simulink library "tramontina_database_RCU_Comissionamentolib"  (R2024a)
settings: Solver=VariableStepAuto  StartTime=0.0  StopTime=10.0  RelTol=1e-3
libraries: canmsglib x4, simulink x1
settings Model: Creator=matlab.cut  LastModifiedBy=matlab.cut

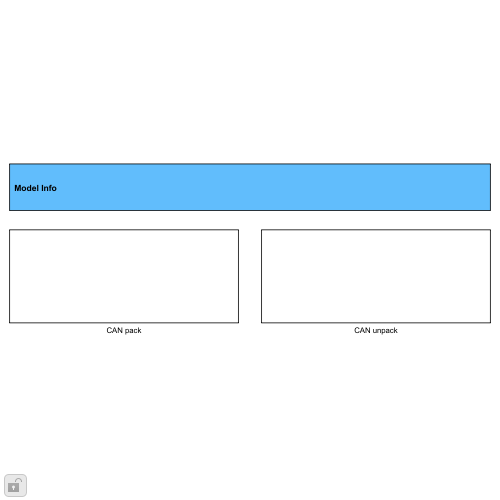
[thumbnail: Simulink's stored preview of the top-level diagram]
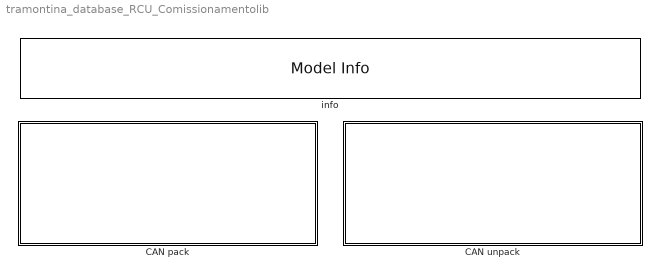
== system tramontina_database_RCU_Comissionamentolib ==
  CAN pack : Subsystem
  CAN unpack : Subsystem
  info : simulink/Model-Wide Utilities/Model Info  Frame=on  DisplayStringWithTags=SPEEDGOAT CAN Database Library for: tramontina_database_RCU_Comissionamento  HorizontalTextAlignment=Left  LeftAlignmentValue=0.01

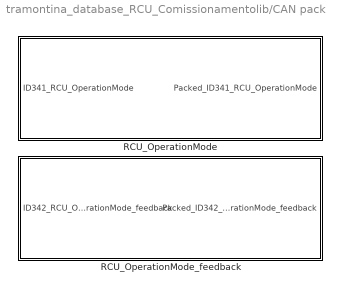
== system tramontina_database_RCU_Comissionamentolib/CAN pack ==
  RCU_OperationMode : Subsystem
  RCU_OperationMode_feedback : Subsystem

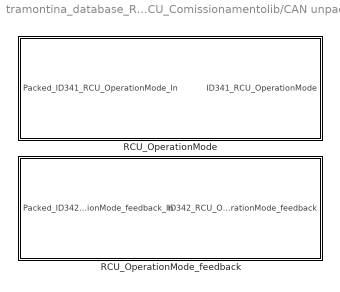
== system tramontina_database_RCU_Comissionamentolib/CAN unpack ==
  RCU_OperationMode : Subsystem
  RCU_OperationMode_feedback : Subsystem

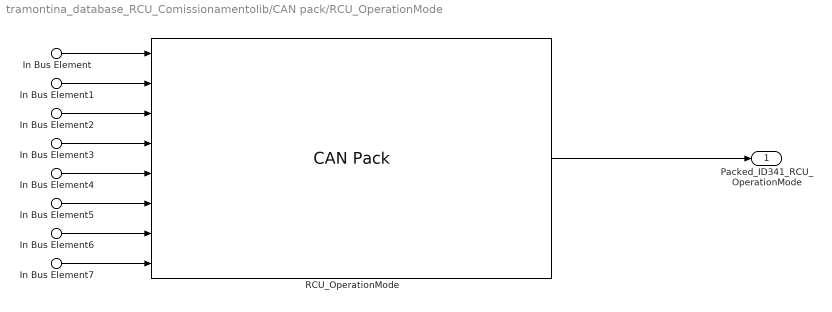
== system tramontina_database_RCU_Comissionamentolib/CAN pack/RCU_OperationMode ==
  In Bus Element : Inport  PortName=ID341_RCU_OperationMode  Element=rcu_front_LeftRigth
  In Bus Element1 : Inport  PortName=ID341_RCU_OperationMode  Element=rcu_front_LoadUnload
  In Bus Element2 : Inport  PortName=ID341_RCU_OperationMode  Element=rcu_front_Run
  In Bus Element3 : Inport  PortName=ID341_RCU_OperationMode  Element=rcu_front_isMoving
  In Bus Element4 : Inport  PortName=ID341_RCU_OperationMode  Element=rcu_rear_LeftRigth
  In Bus Element5 : Inport  PortName=ID341_RCU_OperationMode  Element=rcu_rear_LoadUnload
  In Bus Element6 : Inport  PortName=ID341_RCU_OperationMode  Element=rcu_rear_Run
  In Bus Element7 : Inport  PortName=ID341_RCU_OperationMode  Element=rcu_rear_isMoving
  RCU_OperationMode : canmsglib/CAN Pack  CANdbFile=C:\Users\matlab.cut\Desktop\matlab\AMR_tramontina\Data\DBCFiles\tramontina_database_RCU_Comissionamento.dbc  MsgList=RCU_OperationMode  MsgName=RCU_OperationMode  MsgIDType=Standard (11-bit identifier)  MsgIdentifier=341  MsgLength=8  Remote=off  ApplyMinMax=off  BusOutput=on  SignalInfo={'rcu_front_LeftRigth','1','1','LE','unsigned','Standard','0','1','0','-Inf','Inf';'rcu_front_LoadUnload','0','1','LE','unsigned','Standard','0','1','0','-Inf','Inf';'rcu_front_Run','2','1','LE','unsigned','Standard','0','1','0','-Inf','Inf';'rcu_front_isMoving','3','1','LE','unsigned','Standard','0','1','0','-Inf','Inf';'rcu_rear_LeftRigth','9','1','LE','unsigned','Standard','0','1','0','-Inf','Inf';'rcu_rear_LoadUnload','8','1','LE','unsigned','Standard','0','1','0','-Inf','Inf';'rcu_rear_Run','10','1','LE','unsigned','Standard','0','1','0','-Inf','Inf';'rcu_rear_isMoving','11','1','LE','unsigned','Standard','0','1','0','-Inf','Inf'}
      settings: DataFormat=manually specified signals
  Packed_ID341_RCU_OperationMode : Outport
  wires:
  RCU_OperationMode/1 -> Packed_ID341_RCU_OperationMode/1
  In Bus Element/1 -> RCU_OperationMode/1
  In Bus Element1/1 -> RCU_OperationMode/2
  In Bus Element2/1 -> RCU_OperationMode/3
  In Bus Element3/1 -> RCU_OperationMode/4
  In Bus Element4/1 -> RCU_OperationMode/5
  In Bus Element5/1 -> RCU_OperationMode/6
  In Bus Element6/1 -> RCU_OperationMode/7
  In Bus Element7/1 -> RCU_OperationMode/8

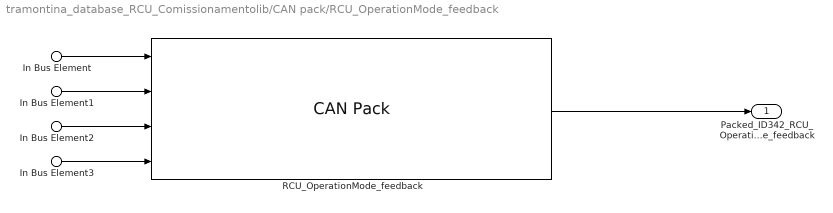
== system tramontina_database_RCU_Comissionamentolib/CAN pack/RCU_OperationMode_feedback ==
  In Bus Element : Inport  PortName=ID342_RCU_OperationMode_feedback  Element=rcu_front_LeftRigth_feedback
  In Bus Element1 : Inport  PortName=ID342_RCU_OperationMode_feedback  Element=rcu_front_LoadUnload_feedback
  In Bus Element2 : Inport  PortName=ID342_RCU_OperationMode_feedback  Element=rcu_front_Run_feedback
  In Bus Element3 : Inport  PortName=ID342_RCU_OperationMode_feedback  Element=rcu_front_isMoving_feedback
  RCU_OperationMode_feedback : canmsglib/CAN Pack  CANdbFile=C:\Users\matlab.cut\Desktop\matlab\AMR_tramontina\Data\DBCFiles\tramontina_database_RCU_Comissionamento.dbc  MsgList=RCU_OperationMode_feedback  MsgName=RCU_OperationMode_feedback  MsgIDType=Standard (11-bit identifier)  MsgIdentifier=342  MsgLength=8  Remote=off  ApplyMinMax=off  BusOutput=on  SignalInfo={'rcu_front_LeftRigth_feedback','1','1','LE','unsigned','Standard','0','1','0','-Inf','Inf';'rcu_front_LoadUnload_feedback','0','1','LE','unsigned','Standard','0','1','0','-Inf','Inf';'rcu_front_Run_feedback','2','1','LE','unsigned','Standard','0','1','0','-Inf','Inf';'rcu_front_isMoving_feedback','3','1','LE','unsigned','Standard','0','1','0','-Inf','Inf'}
      settings: DataFormat=manually specified signals
  Packed_ID342_RCU_OperationMode_feedback : Outport
  wires:
  RCU_OperationMode_feedback/1 -> Packed_ID342_RCU_OperationMode_feedback/1
  In Bus Element/1 -> RCU_OperationMode_feedback/1
  In Bus Element1/1 -> RCU_OperationMode_feedback/2
  In Bus Element2/1 -> RCU_OperationMode_feedback/3
  In Bus Element3/1 -> RCU_OperationMode_feedback/4

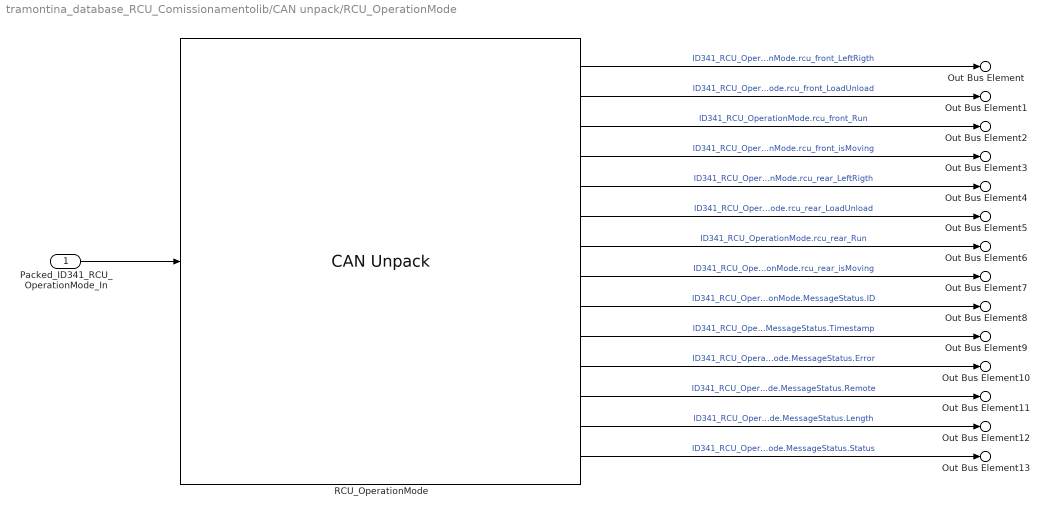
== system tramontina_database_RCU_Comissionamentolib/CAN unpack/RCU_OperationMode ==
  Packed_ID341_RCU_OperationMode_In : Inport
  RCU_OperationMode : canmsglib/CAN Unpack  CANdbFile=C:\Users\matlab.cut\Desktop\matlab\AMR_tramontina\Data\DBCFiles\tramontina_database_RCU_Comissionamento.dbc  MsgList=RCU_OperationMode  MsgName=RCU_OperationMode  MsgIDType=Standard (11-bit identifier)  MsgIdentifier=341  MsgLength=8  SignalInfo={'rcu_front_LeftRigth','1','1','LE','unsigned','Standard','0','1','0','-Inf','Inf';'rcu_front_LoadUnload','0','1','LE','unsigned','Standard','0','1','0','-Inf','Inf';'rcu_front_Run','2','1','LE','unsigned','Standard','0','1','0','-Inf','Inf';'rcu_front_isMoving','3','1','LE','unsigned','Standard','0','1','0','-Inf','Inf';'rcu_rear_LeftRigth','9','1','LE','unsigned','Standard','0','1','0','-Inf','Inf';'rcu_rear_LoadUnload','8','1','LE','unsigned','Standard','0','1','0','-Inf','Inf';'rcu_rear_Run','10','1','LE','unsigned','Standard','0','1','0','-Inf','Inf';'rcu_rear_isMoving','11','1','LE','unsigned','Standard','0','1','0','-Inf','Inf'}  IDPort=on  TimestampPort=on  ErrorPort=on  RemotePort=on  LengthPort=on  StatusPort=on  ApplyMinMax=off
  Out Bus Element : Outport  PortName=ID341_RCU_OperationMode  Element=rcu_front_LeftRigth
  Out Bus Element1 : Outport  PortName=ID341_RCU_OperationMode  Element=rcu_front_LoadUnload
  Out Bus Element2 : Outport  PortName=ID341_RCU_OperationMode  Element=rcu_front_Run
  Out Bus Element3 : Outport  PortName=ID341_RCU_OperationMode  Element=rcu_front_isMoving
  Out Bus Element4 : Outport  PortName=ID341_RCU_OperationMode  Element=rcu_rear_LeftRigth
  Out Bus Element5 : Outport  PortName=ID341_RCU_OperationMode  Element=rcu_rear_LoadUnload
  Out Bus Element6 : Outport  PortName=ID341_RCU_OperationMode  Element=rcu_rear_Run
  Out Bus Element7 : Outport  PortName=ID341_RCU_OperationMode  Element=rcu_rear_isMoving
  Out Bus Element8 : Outport  PortName=ID341_RCU_OperationMode  Element=MessageStatus.ID
  Out Bus Element9 : Outport  PortName=ID341_RCU_OperationMode  Element=MessageStatus.Timestamp
  Out Bus Element10 : Outport  PortName=ID341_RCU_OperationMode  Element=MessageStatus.Error
  Out Bus Element11 : Outport  PortName=ID341_RCU_OperationMode  Element=MessageStatus.Remote
  Out Bus Element12 : Outport  PortName=ID341_RCU_OperationMode  Element=MessageStatus.Length
  Out Bus Element13 : Outport  PortName=ID341_RCU_OperationMode  Element=MessageStatus.Status
  wires:
  Packed_ID341_RCU_OperationMode_In/1 -> RCU_OperationMode/1
  RCU_OperationMode/1 -> Out Bus Element/1  "ID341_RCU_OperationMode.rcu_front_LeftRigth"
  RCU_OperationMode/2 -> Out Bus Element1/1  "ID341_RCU_OperationMode.rcu_front_LoadUnload"
  RCU_OperationMode/3 -> Out Bus Element2/1  "ID341_RCU_OperationMode.rcu_front_Run"
  RCU_OperationMode/4 -> Out Bus Element3/1  "ID341_RCU_OperationMode.rcu_front_isMoving"
  RCU_OperationMode/5 -> Out Bus Element4/1  "ID341_RCU_OperationMode.rcu_rear_LeftRigth"
  RCU_OperationMode/6 -> Out Bus Element5/1  "ID341_RCU_OperationMode.rcu_rear_LoadUnload"
  RCU_OperationMode/7 -> Out Bus Element6/1  "ID341_RCU_OperationMode.rcu_rear_Run"
  RCU_OperationMode/8 -> Out Bus Element7/1  "ID341_RCU_OperationMode.rcu_rear_isMoving"
  RCU_OperationMode/9 -> Out Bus Element8/1  "ID341_RCU_OperationMode.MessageStatus.ID"
  RCU_OperationMode/10 -> Out Bus Element9/1  "ID341_RCU_OperationMode.MessageStatus.Timestamp"
  RCU_OperationMode/11 -> Out Bus Element10/1  "ID341_RCU_OperationMode.MessageStatus.Error"
  RCU_OperationMode/12 -> Out Bus Element11/1  "ID341_RCU_OperationMode.MessageStatus.Remote"
  RCU_OperationMode/13 -> Out Bus Element12/1  "ID341_RCU_OperationMode.MessageStatus.Length"
  RCU_OperationMode/14 -> Out Bus Element13/1  "ID341_RCU_OperationMode.MessageStatus.Status"

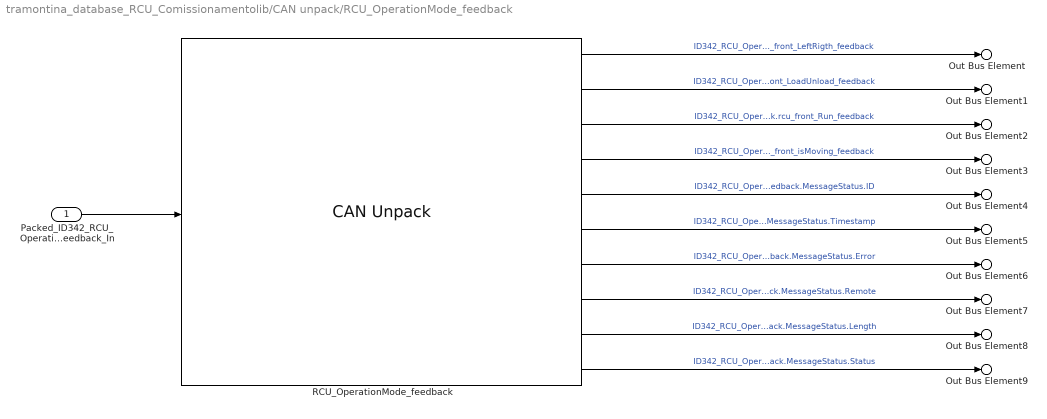
== system tramontina_database_RCU_Comissionamentolib/CAN unpack/RCU_OperationMode_feedback ==
  Packed_ID342_RCU_OperationMode_feedback_In : Inport
  RCU_OperationMode_feedback : canmsglib/CAN Unpack  CANdbFile=C:\Users\matlab.cut\Desktop\matlab\AMR_tramontina\Data\DBCFiles\tramontina_database_RCU_Comissionamento.dbc  MsgList=RCU_OperationMode_feedback  MsgName=RCU_OperationMode_feedback  MsgIDType=Standard (11-bit identifier)  MsgIdentifier=342  MsgLength=8  SignalInfo={'rcu_front_LeftRigth_feedback','1','1','LE','unsigned','Standard','0','1','0','-Inf','Inf';'rcu_front_LoadUnload_feedback','0','1','LE','unsigned','Standard','0','1','0','-Inf','Inf';'rcu_front_Run_feedback','2','1','LE','unsigned','Standard','0','1','0','-Inf','Inf';'rcu_front_isMoving_feedback','3','1','LE','unsigned','Standard','0','1','0','-Inf','Inf'}  IDPort=on  TimestampPort=on  ErrorPort=on  RemotePort=on  LengthPort=on  StatusPort=on  ApplyMinMax=off
  Out Bus Element : Outport  PortName=ID342_RCU_OperationMode_feedback  Element=rcu_front_LeftRigth_feedback
  Out Bus Element1 : Outport  PortName=ID342_RCU_OperationMode_feedback  Element=rcu_front_LoadUnload_feedback
  Out Bus Element2 : Outport  PortName=ID342_RCU_OperationMode_feedback  Element=rcu_front_Run_feedback
  Out Bus Element3 : Outport  PortName=ID342_RCU_OperationMode_feedback  Element=rcu_front_isMoving_feedback
  Out Bus Element4 : Outport  PortName=ID342_RCU_OperationMode_feedback  Element=MessageStatus.ID
  Out Bus Element5 : Outport  PortName=ID342_RCU_OperationMode_feedback  Element=MessageStatus.Timestamp
  Out Bus Element6 : Outport  PortName=ID342_RCU_OperationMode_feedback  Element=MessageStatus.Error
  Out Bus Element7 : Outport  PortName=ID342_RCU_OperationMode_feedback  Element=MessageStatus.Remote
  Out Bus Element8 : Outport  PortName=ID342_RCU_OperationMode_feedback  Element=MessageStatus.Length
  Out Bus Element9 : Outport  PortName=ID342_RCU_OperationMode_feedback  Element=MessageStatus.Status
  wires:
  Packed_ID342_RCU_OperationMode_feedback_In/1 -> RCU_OperationMode_feedback/1
  RCU_OperationMode_feedback/1 -> Out Bus Element/1  "ID342_RCU_OperationMode_feedback.rcu_front_LeftRigth_feedback"
  RCU_OperationMode_feedback/2 -> Out Bus Element1/1  "ID342_RCU_OperationMode_feedback.rcu_front_LoadUnload_feedback"
  RCU_OperationMode_feedback/3 -> Out Bus Element2/1  "ID342_RCU_OperationMode_feedback.rcu_front_Run_feedback"
  RCU_OperationMode_feedback/4 -> Out Bus Element3/1  "ID342_RCU_OperationMode_feedback.rcu_front_isMoving_feedback"
  RCU_OperationMode_feedback/5 -> Out Bus Element4/1  "ID342_RCU_OperationMode_feedback.MessageStatus.ID"
  RCU_OperationMode_feedback/6 -> Out Bus Element5/1  "ID342_RCU_OperationMode_feedback.MessageStatus.Timestamp"
  RCU_OperationMode_feedback/7 -> Out Bus Element6/1  "ID342_RCU_OperationMode_feedback.MessageStatus.Error"
  RCU_OperationMode_feedback/8 -> Out Bus Element7/1  "ID342_RCU_OperationMode_feedback.MessageStatus.Remote"
  RCU_OperationMode_feedback/9 -> Out Bus Element8/1  "ID342_RCU_OperationMode_feedback.MessageStatus.Length"
  RCU_OperationMode_feedback/10 -> Out Bus Element9/1  "ID342_RCU_OperationMode_feedback.MessageStatus.Status"
